simulink model "battery_project_more_constraints"  (R2023b)
settings: Solver=VariableStepAuto  StartTime=0.0  StopTime=600  RelTol=1e-3
model workspace (MAT data in the model file):
  A = Simulink.Parameter
  A.DataType = 'auto'
  A.Complexity = 'real'
  A.Dimensions = [0 0]
  B = 1
  C = 1
  D = 1
values from neighbouring files (symbols this model uses):
  A_mat = [0, 0; 0, - 1 / (C*R1)]    [state_space_1_vars.m]
  B_mat = [1/Q; 1/C]    [state_space_1_vars.m]
  C_mat = [1, 0; 0, 1; p_1 + p_2 + 3*p_3 / 4, 0]    [state_space_1_vars.m]
  D_dummy = [0; 0; 0]    [state_space_1_vars.m]
  p_0 = 3.4707    [state_space_1_vars.m]
  p_1 = 1.6112    [state_space_1_vars.m]
  p_2 = -2.6287    [state_space_1_vars.m]
  p_3 = 1.7175    [state_space_1_vars.m]
  x0 = [z0, V_c0]    [state_space_1_vars.m]
libraries: mpclib x1
settings Model: Creator=Teama  LastModifiedBy=Teama
settings OptimizationCC: ReuseModelBlockBuffer=off
settings DebuggingCC: AlgebraicLoopMsg=none

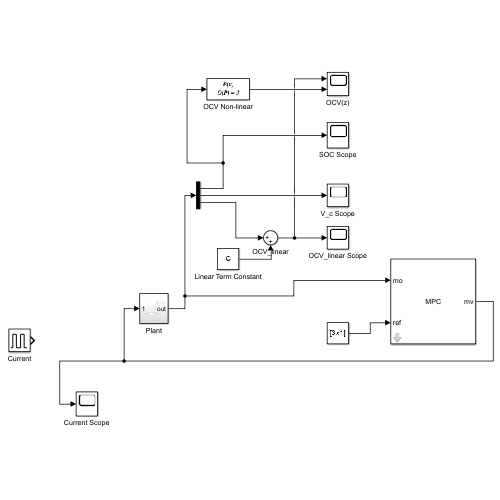
[thumbnail: Simulink's stored preview of the top-level diagram]
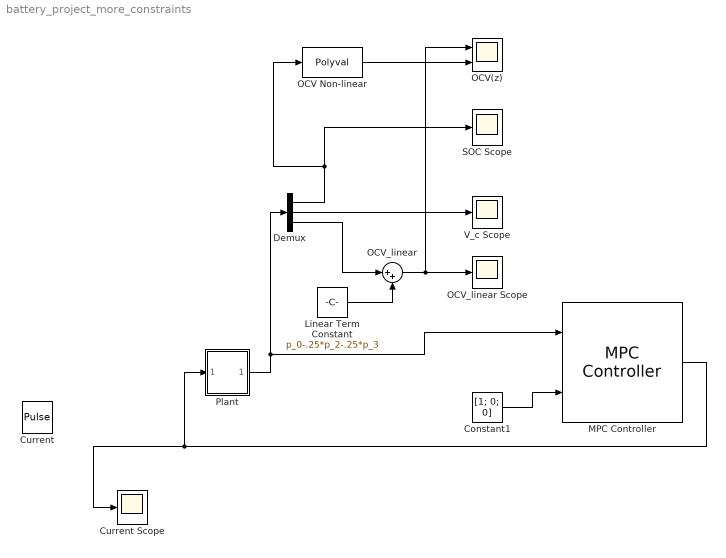
== system battery_project_more_constraints ==
  Constant1 : Constant  Value=[1; 0; 0]
  Current : DiscretePulseGenerator  PulseType=Time based  Amplitude=-5  Period=40  PulseWidth=50
  Current Scope : Scope
  Demux : Demux  Outputs=3
  Linear Term Constant : Constant  Value=p_0-.25*p_2-.25*p_3
  MPC Controller : mpclib/MPC Controller  SCDEnableBlockLinearizationSpecification=on  mpcobj=mpc1  is_multiple=0  enable_value=0  return_u0=off  updateMPCinCallerWorkspace=on  md_inport=off  mv_inport=off  uref_inport=off  return_cost=off  return_mvseq=off  return_qpstatus=off  return_xseq=off  return_state=off  return_ovseq=off  state_inport=off  umin_inport=off  umax_inport=off  ymin_inport=off  ymax_inport=off  cc_inport=off  ywt_inport=off  uwt_inport=off  duwt_inport=off  rhoeps_inport=off  pm_inport=off  MaximumP=10  HorizonChoice=FixedHorizon  n_ts=1  n_p=10  n_mv=1  n_md=0  n_ud=0  n_mo=3  n_uo=0  BlockDataType=double  SampleTimeInherited=off  switch_inport=off
  OCV Non-linear : Polyval  Coefs=[p_3, p_2, p_1, p_0]
  OCV(z) : Scope  NumInputPorts=2
  OCV_linear : Sum  Inputs=|++
  OCV_linear Scope : Scope
  Plant : Subsystem
  SOC Scope : Scope
  V_c Scope : Scope
  wires:
  Plant/1(out) -> Demux/1, MPC Controller/1
  OCV Non-linear/1 -> OCV(z)/2
  Demux/1 -> SOC Scope/1, OCV Non-linear/1
  Demux/2 -> V_c Scope/1
  Demux/3 -> OCV_linear/1
  Linear Term Constant/1 -> OCV_linear/2
  OCV_linear/1 -> OCV(z)/1, OCV_linear Scope/1
  MPC Controller/1 -> Current Scope/1, Plant/1(In1)
  Constant1/1 -> MPC Controller/2

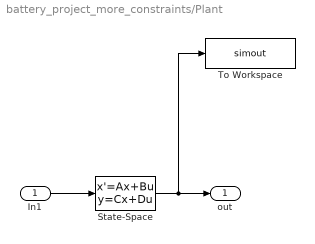
== system battery_project_more_constraints/Plant ==
  In1 : Inport
  State-Space : StateSpace  A=A_mat  B=B_mat  C=C_mat  D=D_dummy  InitialCondition=x0
  To Workspace : ToWorkspace  VariableName=simout  SaveFormat=Timeseries  SampleTime=-1
  out : Outport
  wires:
  State-Space/1 -> out/1, To Workspace/1
  In1/1 -> State-Space/1
